simulink model "fault"  (R2024b)
settings: Solver=ode45  StartTime=0.0  StopTime=0.6  RelTol=1e-3
libraries: spsThreePhaseFaultLib x6, spsDistributedParametersLineLib x2, spsThreePhaseSourceLib x2, spsGroundLib x1, spsThreePhaseParallelRLCLoadLib x1, spsThreePhaseVIMeasurementLib x1, spsThreePhaseTransformer12TerminalsLib x1, spspowerguiLib x1
settings Model: Creator=abisek  LastModifiedBy=abisek
settings SolverCC: AlgebraicLoopSolver=TrustRegion  MaxZcPerStep=1
settings DataIOCC: LimitDataPoints=on  SaveOperatingPoint=on  SaveFormat=Array  ReturnWorkspaceOutputs=off
settings DebuggingCC: SolverPrmCheckMsg=warning  UnconnectedInputMsg=warning  UnconnectedOutputMsg=warning  UnconnectedLineMsg=warning  StateNameClashWarn=warning  SymbolicDimsDataTypeCodeGenerationDiagnostic=none
settings ModelReferenceCC: EnableRefExpFcnMdlSchedulingChecks=on  PropagateSignalLabelsOutOfModel=off
settings SFSimCC: CustomCodeUndefinedFunction=UseInterfaceOnly
settings RTWCC: GPUComputeCapability=3.5  DLArmComputeVersion=19.05
settings GRTTargetCC: TargetLangStandard=C89/C90 (ANSI)
settings SimscapeCC: SimscapeNormalizeSystem=off  SimscapeLogDataHistory=10000

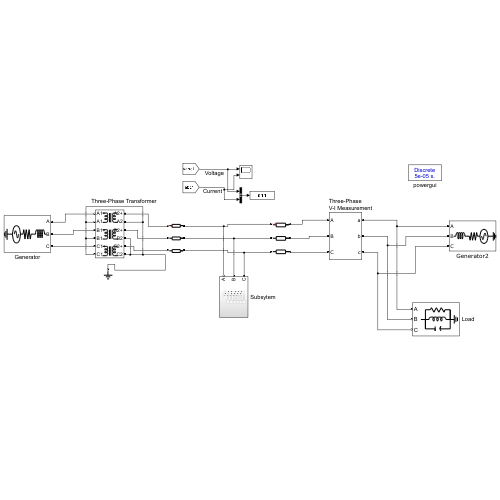
[thumbnail: Simulink's stored preview of the top-level diagram]
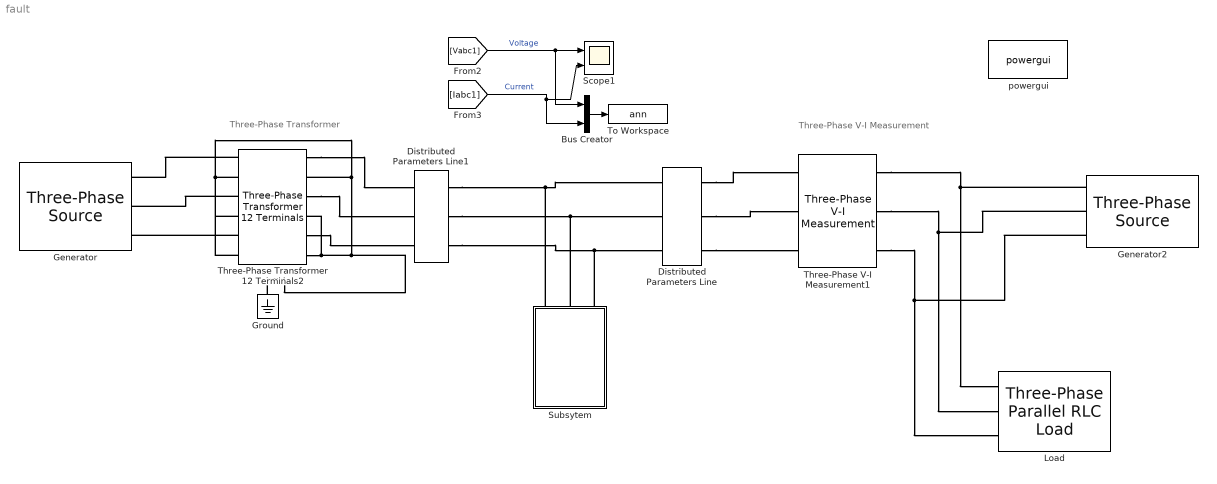
== system fault ==
  note: Three-Phase
      | V-I Measurement
  note: Three-Phase Transformer
  Bus Creator : BusCreator  Inputs=2
  Distributed Parameters Line : spsDistributedParametersLineLib/Distributed Parameters Line  Phases=3  Length=33  Frequency=50  Resistance=[0.0132 0.132]  Inductance="[0.9337e-3  4.1264e-3]"  Capacitance=[12.74e-9 7.751e-9]  x1=[-0.0002 -7.76954668176518e-12 0 0;-0.00015 -7.87646396901458e-12 5974.88340798078 -10563.6292091691;-0.0001 -7.98143785663768e-12 6140.07257739521 -10468.4766108587;-5e-05 -8.08444244389848e-12 6303.74677577704 -10370.7410725876]  x2=[-0.0002 -1.01560231735665e-11 0 0;-0.00015 -1.01218647402771e-11 5358.85846556688 -10536.0998734294;-0.0001 -1.00852088883198e-11 5523.69122043783 -10450.6267705872;-5e-05 -1.00460646619774e-11 5687.16108715292 -10362.5751319655]  x3=[-0.0002 -2.48027199467017e-13 0 0;-0.00015 -2.47656360151501e-13 21.327638612534 24.2331785585823;-0.0001 -2.47224415334879e-13 20.9443692495927 24.565188958681;-5e-05 -2.46731471593072e-13 20.5559321769363 24.8911382659809]  x4=[-0.0002 2.00367175354438e-13 0 0;-0.00015 2.01711156359462e-13 19.0947396805588 -102.826680254378;-0.0001 2.03005368154923e-13 20.7075153047877 -102.514067646866;-5e-05 2.04249491413427e-13 22.3151816594683 -102.176161227114]  x5=0.000186628717108595  V1=[2.547e-09 1.32e+05 1.32e+05;314.2 314.2 314.2;-0.1043 0.8095 -0.7613]  V2=[2.522e-09 1.32e+05 1.32e+05;314.2 314.2 314.2;-0.1193 0.8007 -0.7701]  I1=[2.615e-12 367.2 367.2;314.2 314.2 314.2;-0.5343 0.7771 -0.7937]  I2=[5.144e-12 607 607;314.2 314.2 314.2;-0.488 0.7934 -0.7774]  nHarmo=1  Measurements=None  Decoupling=off  VsMag0=0  VrMag0=0  VsAngle0=0  VrAngle0=0  IsMag0=0  IrMag0=0  IsAngle0=0  IrAngle0=0
      settings: LibrarySourceBlock=sps_lib/Power Grid Elements/Distributed Parameters Line
  Distributed Parameters Line1 : spsDistributedParametersLineLib/Distributed Parameters Line  Phases=3  Length=33  Frequency=50  Resistance=[0.0132 0.132]  Inductance="[0.9337e-3  4.1264e-3]"  Capacitance=[12.74e-9 7.751e-9]  x1=[-0.0002 4.28307336251101e-13 0 0;-0.00015 3.21323005048107e-13 6584.50685105916 -10576.991236017;-0.0001 2.14259392201677e-13 6749.83069433792 -10472.2614404053;-5e-05 1.07142914056253e-13 6913.48911789273 -10364.947770983]  x2=[-0.0002 -7.76954668176518e-12 0 0;-0.00015 -7.87646396901458e-12 5974.88340798078 -10563.6292091691;-0.0001 -7.98143785663768e-12 6140.07257739521 -10468.4766108587;-5e-05 -8.08444244389848e-12 6303.74677577704 -10370.7410725876]  x3=[-0.0002 4.80522780531151e-14 0 0;-0.00015 4.40242849583402e-14 22.1458230758777 23.4183852653392;-0.0001 3.99854295300013e-14 21.7752509923501 23.7633476674497;-5e-05 3.59367082952408e-14 21.3993061914702 24.1024468191019]  x4=[-0.0002 1.23595060927633e-13 0 0;-0.00015 1.24621782580923e-13 22.7957759953166 -102.243636593161;-0.0001 1.25617755674116e-13 24.3989369800867 -101.872962562521;-5e-05 1.26582734465755e-13 25.9960778922461 -101.477152902727]  x5=0.000186628717108595  V1=[2.618e-09 1.319e+05 1.319e+05;314.2 314.2 314.2;-0.1003 0.8184 -0.7524]  V2=[2.549e-09 1.32e+05 1.32e+05;314.2 314.2 314.2;-0.1043 0.8095 -0.7613]  I1=[2.387e-12 367.3 367.3;314.2 314.2 314.2;0.1434 0.7414 -0.8294]  I2=[6.175e-12 607.4 607.4;314.2 314.2 314.2;-0.4569 0.8292 -0.7416]  nHarmo=1  Measurements=None  Decoupling=off  VsMag0=0  VrMag0=0  VsAngle0=0  VrAngle0=0  IsMag0=0  IrMag0=0  IsAngle0=0  IrAngle0=0
      settings: LibrarySourceBlock=sps_lib/Power Grid Elements/Distributed Parameters Line
  Generator : spsThreePhaseSourceLib/Three-Phase Source  InternalConnection=Yg  VoltagePhases=off  Voltage=11e3  PhaseAngle=0  Voltage_phases=[25e3 25e3 25e3]/sqrt(3)  PhaseAngles_phases=[0 -120 +120]  Frequency=50  NonIdealSource=on  SpecifyImpedance=off  Resistance=12  Inductance=16.58e-3  ShortCircuitLevel=20e6  BaseVoltage=11e3  XRratio=7  BusType=PV  Pref=50e6  Qref=0  Prefabc=[10e3, 10e3, 10e3]  Qrefabc=[0, 0, 0]  Qmin=-inf  Qmax=inf
  Generator2 : spsThreePhaseSourceLib/Three-Phase Source  InternalConnection=Yg  VoltagePhases=off  Voltage=11e3  PhaseAngle=0  Voltage_phases=[25e3 25e3 25e3]/sqrt(3)  PhaseAngles_phases=[0 -120 +120]  Frequency=50  NonIdealSource=on  SpecifyImpedance=off  Resistance=12  Inductance=16.58e-3  ShortCircuitLevel=20e6  BaseVoltage=11e3  XRratio=7  BusType=PV  Pref=20e6  Qref=0  Prefabc=[10e3, 10e3, 10e3]  Qrefabc=[0, 0, 0]  Qmin=-inf  Qmax=inf
  Ground : spsGroundLib/Ground  LConnTagsString=a
  Load : spsThreePhaseParallelRLCLoadLib/Three-Phase Parallel RLC Load  LConnTagsString=A|B|C  Configuration=Y (grounded)  NominalVoltage=1000  Vabc=[1e3 1e3 1e3]  Vabcp=[1e3 1e3 1e3]  NominalFrequency=60  UnbalancedPower=off  ActivePower=100  InductivePower=10  CapacitivePower=10  Pabc=[10e3 9e3 11e3]  QLabc=[100 90 110]  QCabc=[100 90 110]  Pabcp=[10e3 9e3 11e3]  QLabcp=[100 90 110]  QCabcp=[100 90 110]  Measurements=None  LoadType=constant Z
  Scope1 : Scope  NumInputPorts=2
  Subsytem : Subsystem
  Three-Phase V-I Measurement1 : spsThreePhaseVIMeasurementLib/Three-Phase V-I Measurement  VoltageMeasurement=phase-to-phase  SetLabelV=on  LabelV=Vabc1  Vpu=off  VpuLL=on  CurrentMeasurement=yes  SetLabelI=on  LabelI=Iabc1  Ipu=off  Pbase=100e6  Vbase=11e3  OutputType=Complex  PhasorSimulation=off  PSBequivalent=0
  Three-Phase Transformer 12 Terminals2 : spsThreePhaseTransformer12TerminalsLib/Three-Phase Transformer 12 Terminals  RatedPower=[100e6 50]  Winding1="[ 11e3 0.002  0.05 ]"  Winding2=[ 132e3 0.002 0.05]  RmXm=[ 200 200 ]
      settings: LibrarySourceBlock=|
      | sps_lib/Power Grid Elements/Three-Phase Transformer
      | 12 Terminals
  To Workspace : ToWorkspace  VariableName=ann  SaveFormat=Structure With Time  SampleTime=-1
  "powergui " : spspowerguiLib/powergui  Priority=1  SimulationMode=Discrete  SampleTime=50e-6  frequency=60  Iterations=50  frequencyindice=50  Pbase=100e6  ErrMax=1e-4  UnitsV=kV  UnitsW=MW  buscounter=0  FunctionMessages=off  echomessages=off  EnableUseOfTLC=off  CurrentSourceSwitches=off  DisableSnubberDevices=off  DisableRonSwitches=off  DisableVfSwitches=off  DisplayEquations=off  AutomaticDiscreteSolvers=off  SolverType=Tustin/Backward Euler (TBE)  Interpol=off  ExternalGateDelay=off  methode=off  Ts=100  x0status=blocks  SPID=on  SwTol=0  HookPort=off  NonlinearTolerance=1e-4  nMaxIteration=100  ContinueOnMaxIteration=off  RestoreLinks=warning  ResistiveCurrentMeasurement=off  Frange=[0:2:500]  Ylog=off  Xlog=on  ShowGrid=off  save=off  variable=ZData  structure=0  ZoomFFT=off  StartTime=0.0  cycles=1  DisplayStyle=1  fundamental=60  FreqAxis=off  MaxFrequency=1000  frequencyindicesteady=1  RmsSteady=1  display=off
  wires:
  [Iabc1] -> Bus Creator/2, Scope1/2  "Current"
  Bus Creator/1 -> To Workspace/1
  [Vabc1] -> Bus Creator/1, Scope1/1  "Voltage"
  connections:
  Three-Phase Transformer 12 Terminals2/LConn2 -- Three-Phase Transformer 12 Terminals2/LConn6 -- Three-Phase Transformer 12 Terminals2/LConn4 -- Three-Phase Transformer 12 Terminals2/RConn4 -- Three-Phase Transformer 12 Terminals2/RConn6 -- Ground/LConn1 -- Three-Phase Transformer 12 Terminals2/RConn2
  Three-Phase Transformer 12 Terminals2/LConn1 -- Generator/RConn1
  Three-Phase Transformer 12 Terminals2/LConn3 -- Generator/RConn2
  Three-Phase Transformer 12 Terminals2/LConn5 -- Generator/RConn3
  Three-Phase V-I Measurement1/RConn1 -- Generator2/RConn1 -- Load/LConn1
  Three-Phase V-I Measurement1/RConn2 -- Generator2/RConn2 -- Load/LConn2
  Three-Phase V-I Measurement1/RConn3 -- Generator2/RConn3 -- Load/LConn3
  Three-Phase Transformer 12 Terminals2/RConn5 -- Distributed Parameters Line1/LConn3
  Three-Phase Transformer 12 Terminals2/RConn3 -- Distributed Parameters Line1/LConn2
  Three-Phase Transformer 12 Terminals2/RConn1 -- Distributed Parameters Line1/LConn1
  Distributed Parameters Line/RConn1 -- Three-Phase V-I Measurement1/LConn1
  Distributed Parameters Line/RConn2 -- Three-Phase V-I Measurement1/LConn2
  Distributed Parameters Line/RConn3 -- Three-Phase V-I Measurement1/LConn3
  Distributed Parameters Line1/RConn1 -- Subsytem/LConn1 -- Distributed Parameters Line/LConn1
  Distributed Parameters Line1/RConn2 -- Subsytem/LConn2 -- Distributed Parameters Line/LConn2
  Distributed Parameters Line1/RConn3 -- Subsytem/LConn3 -- Distributed Parameters Line/LConn3

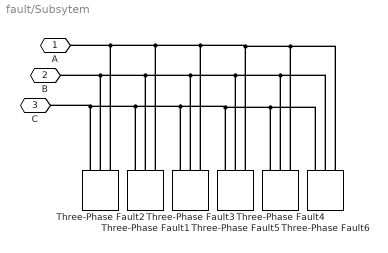
== system fault/Subsytem ==
  Three-Phase Fault1 : spsThreePhaseFaultLib/Three-Phase Fault  InitialStates=0  FaultA=on  FaultB=on  FaultC=off  GroundFault=on  SwitchTimes=[ 0.125 0.175]  External=off  SwitchStatus=NaN  FaultResistance=0.001  GroundResistance=0.001  SnubberResistance=1e6  SnubberCapacitance=inf  Measurements=None
  Three-Phase Fault2 : spsThreePhaseFaultLib/Three-Phase Fault  InitialStates=0  FaultA=on  FaultB=off  FaultC=off  GroundFault=on  SwitchTimes=[ 0.025 0.075]  External=off  SwitchStatus=NaN  FaultResistance=0.001  GroundResistance=0.001  SnubberResistance=1e6  SnubberCapacitance=inf  Measurements=None
  Three-Phase Fault3 : spsThreePhaseFaultLib/Three-Phase Fault  InitialStates=0  FaultA=off  FaultB=on  FaultC=on  GroundFault=off  SwitchTimes=[ 0.225 0.275]  External=off  SwitchStatus=NaN  FaultResistance=0.001  GroundResistance=0.001  SnubberResistance=1e6  SnubberCapacitance=inf  Measurements=None
  Three-Phase Fault4 : spsThreePhaseFaultLib/Three-Phase Fault  InitialStates=0  FaultA=on  FaultB=on  FaultC=on  GroundFault=on  SwitchTimes=[ 0.425 0.475]  External=off  SwitchStatus=NaN  FaultResistance=0.001  GroundResistance=0.001  SnubberResistance=1e6  SnubberCapacitance=inf  Measurements=None
  Three-Phase Fault5 : spsThreePhaseFaultLib/Three-Phase Fault  InitialStates=0  FaultA=on  FaultB=on  FaultC=on  GroundFault=off  SwitchTimes=[ 0.325 0.375]  External=off  SwitchStatus=NaN  FaultResistance=0.001  GroundResistance=0.001  SnubberResistance=1e6  SnubberCapacitance=inf  Measurements=None
  Three-Phase Fault6 : spsThreePhaseFaultLib/Three-Phase Fault  InitialStates=0  FaultA=off  FaultB=off  FaultC=off  GroundFault=off  SwitchTimes=[ 0.525 0.575]  External=off  SwitchStatus=NaN  FaultResistance=0.001  GroundResistance=0.001  SnubberResistance=1e6  SnubberCapacitance=inf  Measurements=None
  A : PMIOPort  Side=Left
  B : PMIOPort  Port=2  Side=Left
  C : PMIOPort  Port=3  Side=Left
  connections:
  Three-Phase Fault2/LConn2 -- Three-Phase Fault6/LConn2 -- Three-Phase Fault4/LConn2 -- Three-Phase Fault5/LConn2 -- Three-Phase Fault3/LConn2 -- Three-Phase Fault1/LConn2 -- B/RConn1
  Three-Phase Fault2/LConn3 -- Three-Phase Fault6/LConn3 -- Three-Phase Fault4/LConn3 -- Three-Phase Fault5/LConn3 -- Three-Phase Fault3/LConn3 -- Three-Phase Fault1/LConn3 -- C/RConn1
  Three-Phase Fault2/LConn1 -- Three-Phase Fault6/LConn1 -- Three-Phase Fault4/LConn1 -- Three-Phase Fault5/LConn1 -- Three-Phase Fault3/LConn1 -- Three-Phase Fault1/LConn1 -- A/RConn1
